simulink model "SOP_test"  (R2018b)
settings: Solver=VariableStepAuto  StartTime=0.0  StopTime=2*5.01*3600  RelTol=1e-3
undefined symbols (not defined in the file): n
settings Model: Creator=Pedro  LastModifiedBy=Pedro

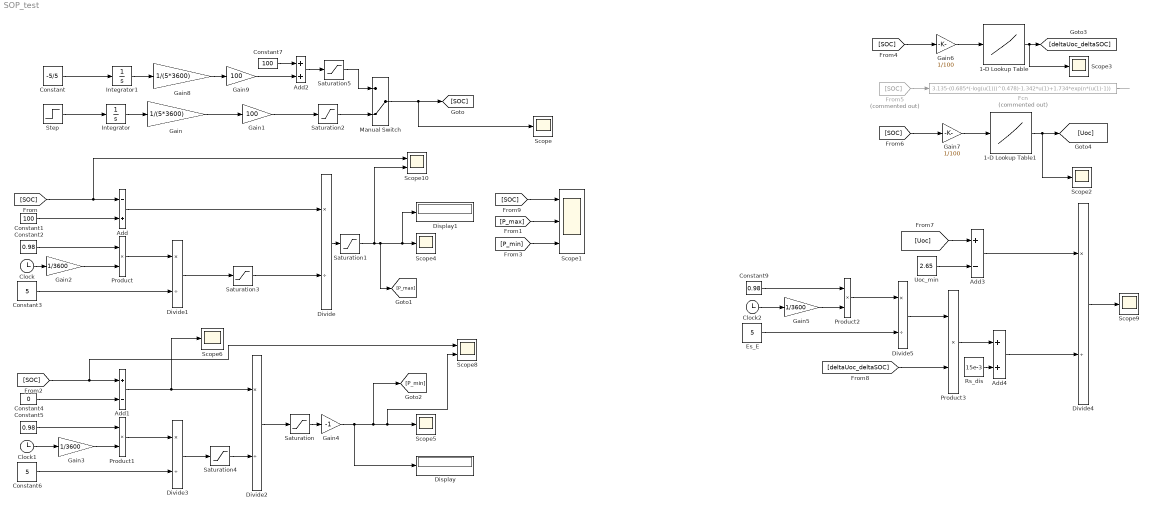
== system SOP_test ==
  1-D Lookup Table : Lookup_n-D  NumberOfTableDimensions=1  BreakpointsSpecification=Even spacing  BreakpointsForDimension1=[0:1]  BreakpointsForDimension1FirstPoint=0.1  BreakpointsForDimension1Spacing=0.1  Table=[6.1,0.5,0.6,0.4,0.4,0.5,0.9,0.1,0.1,0.1]  InternalRulePriority=Speed  RndMeth=Simplest  InputSameDT=on
  1-D Lookup Table1 : Lookup_n-D  NumberOfTableDimensions=1  BreakpointsSpecification=Even spacing  BreakpointsForDimension1=[0:1]  BreakpointsForDimension1FirstPoint=0.1  BreakpointsForDimension1Spacing=0.1  Table=[2.64,3.2,3.25,3.255,3.256,3.257,3.27,3.29,3.3,3.45]  InternalRulePriority=Speed  RndMeth=Simplest  InputSameDT=on
  Add : Sum  Inputs=-+
  Add1 : Sum  Inputs=+-
  Add2 : Sum
  Add3 : Sum  Inputs=+-
  Add4 : Sum
  Clock : Clock
  Clock1 : Clock
  Clock2 : Clock
  Constant : Constant  Value=-5/5
  Constant1 : Constant  Value=100
  Constant2 : Constant  Value=0.98
  Constant3 : Constant  Value=5
  Constant4 : Constant  Value=0
  Constant5 : Constant  Value=0.98
  Constant6 : Constant  Value=5
  Constant7 : Constant  Value=100
  Constant9 : Constant  Value=0.98
  Display : Display
  Display1 : Display
  Divide{,1..5} (6 alike) : Product  Inputs=*/
  Es_E : Constant  Value=5
  Fcn : Fcn  Commented=on  Expr=3.135-(0.685*(-log(u(1)))^0.478)-1.342*u(1)+1.734*exp(n*(u(1)-1))
  From5 : From  Commented=on  GotoTag=SOC
  Gain : Gain  Gain=1/(5*3600)
  Gain1 : Gain  Gain=100
  Gain2 : Gain  Gain=1/3600
  Gain3 : Gain  Gain=1/3600
  Gain4 : Gain  Gain=-1
  Gain5 : Gain  Gain=1/3600
  Gain6 : Gain  Gain=1/100
  Gain7 : Gain  Gain=1/100
  Gain8 : Gain  Gain=1/(5*3600)
  Gain9 : Gain  Gain=100
  Integrator : Integrator
  Integrator1 : Integrator
  Manual Switch : ManualSwitch  CurrentSetting=0
  Product{,1..3} (4 alike) : Product
  "Rs_dis " : Constant  Value=15e-3
  Saturation : Saturate  UpperLimit=5/5  LowerLimit=-inf
  Saturation1 : Saturate  UpperLimit=5/5  LowerLimit=0
  Saturation2 : Saturate  UpperLimit=100  LowerLimit=0
  Saturation3 : Saturate  UpperLimit=inf  LowerLimit=1e-03
  Saturation4 : Saturate  UpperLimit=inf  LowerLimit=1e-02
  Saturation5 : Saturate  UpperLimit=100  LowerLimit=0
  Scope{,2..6,9} (7 alike) : Scope
  Scope1 : Scope  NumInputPorts=3
  Scope10 : Scope  NumInputPorts=2
  Scope8 : Scope  NumInputPorts=2
  Step : Step  Time=5.01*3600  Before=1  After=-1  SampleTime=0
  "Uoc_min " : Constant  Value=2.65
  wires:
  Integrator/1 -> Gain/1
  Gain/1 -> Gain1/1
  [SOC] -> Scope10/1, Add/1
  Constant1/1 -> Add/2
  Add/1 -> Divide/1
  Clock/1 -> Gain2/1
  Constant2/1 -> Product/1
  Gain2/1 -> Product/2
  Divide1/1 -> Saturation3/1
  Product/1 -> Divide1/1
  Constant3/1 -> Divide1/2
  Divide/1 -> Saturation1/1
  Divide3/1 -> Saturation4/1
  Gain4/1 -> Display/1, Scope8/2, Scope5/1, [P_min]
  Constant6/1 -> Divide3/2
  [SOC] -> Scope8/1, Add1/1
  Add1/1 -> Scope6/1, Divide2/1
  Gain3/1 -> Product1/2
  Constant5/1 -> Product1/1
  Clock1/1 -> Gain3/1
  Constant4/1 -> Add1/2
  Product1/1 -> Divide3/1
  [SOC] -> Gain6/1
  1-D Lookup Table/1 -> Scope3/1, [deltaUoc_deltaSOC]
  Gain1/1 -> Saturation2/1
  From5/1 -> Fcn/1
  Fcn/1 -> ?
  [SOC] -> Gain7/1
  "Uoc_min "/1 -> Add3/2
  [Uoc] -> Add3/1
  Add3/1 -> Divide4/1
  Clock2/1 -> Gain5/1
  Es_E/1 -> Divide5/2
  Constant9/1 -> Product2/1
  Gain5/1 -> Product2/2
  Product2/1 -> Divide5/1
  Divide5/1 -> Product3/1
  [deltaUoc_deltaSOC] -> Product3/2
  Product3/1 -> Add4/1
  "Rs_dis "/1 -> Add4/2
  Add4/1 -> Divide4/2
  Divide4/1 -> Scope9/1
  1-D Lookup Table1/1 -> Scope2/1, [Uoc]
  Divide2/1 -> Saturation/1
  Saturation1/1 -> Scope10/2, Display1/1, Scope4/1, [P_max]
  [P_max] -> Scope1/2
  [P_min] -> Scope1/3
  [SOC] -> Scope1/1
  Saturation2/1 -> Manual Switch/2
  Saturation/1 -> Gain4/1
  Saturation3/1 -> Divide/2
  Saturation4/1 -> Divide2/2
  Step/1 -> Integrator/1
  Gain6/1 -> 1-D Lookup Table/1
  Gain7/1 -> 1-D Lookup Table1/1
  Manual Switch/1 -> Scope/1, [SOC]
  Gain8/1 -> Gain9/1
  Add2/1 -> Saturation5/1
  Integrator1/1 -> Gain8/1
  Constant/1 -> Integrator1/1
  Saturation5/1 -> Manual Switch/1
  Gain9/1 -> Add2/2
  Constant7/1 -> Add2/1
